simulink model "autosar_swc_monitor"  (R2021a)
settings: Solver=FixedStepDiscrete  StartTime=0.0  StopTime=10.0  FixedStep=0.02  RelTol=1e-3
PreLoadFcn:
  | Simulink.defineIntEnumType('SensorOption',...
  |     {'Primary', 'Secondary'},...
  |     [0;1],...
  |     'DefaultValue', 'Primary');
  | 
  | SensorSelection = Simulink.Parameter;
  | SensorSelection.Value = SensorOption.Primary;
  | SensorSelection.DataType = 'Enum: SensorOption';
libraries: simulink x1
settings Model: Creator=The MathWorks, Inc.  LastModifiedBy=ASUS
settings SolverCC: AlgebraicLoopSolver=TrustRegion
settings DataIOCC: SaveFormat=StructureWithTime  ReturnWorkspaceOutputs=off
settings OptimizationCC: DefaultParameterBehavior=Inlined  PassReuseOutputArgsAs=Individual arguments  ZeroExternalMemoryAtStartup=off  ZeroInternalMemoryAtStartup=off  EfficientTunableParamExpr=on
settings DebuggingCC: ParameterTunabilityLossMsg=error  SFMachineParentedDataDiag=warning  ArithmeticOperatorsInVariantConditions=warning
settings SFSimCC: SimUseLocalCustomCode=off  MATLABDynamicMemAlloc=off  CustomCodeUndefinedFunction=UseInterfaceOnly
settings RTWCC: Description=AUTOSAR  SystemTargetFile=autosar.tlc  GenCodeOnly=on  TemplateMakefile=ert_default_tmf  GenerateReport=on  RTWUseLocalCustomCode=off  IncludeHyperlinkInReport=on  LaunchReport=on  GenerateTraceInfo=on  GenerateTraceReport=on  GenerateTraceReportSl=on  GenerateTraceReportSf=on  GenerateTraceReportEml=on
settings CodeAppCC: ForceParamTrailComments=on  IgnoreCustomStorageClasses=off  OperatorAnnotations=on  SimulinkDataObjDesc=on  SFDataObjDesc=on  InsertBlockDesc=on
settings STFCustomTargetCC: TargetLangStandard=C99 (ISO)  MultiwordLength=256  ParMdlRefBuildCompliant=on  CompOptLevelCompliant=on  IncludeMdlTerminateFcn=off  CombineOutputUpdateFcns=on  SuppressErrorStatus=on  ERTCustomFileBanners=on  SupportNonFinite=off  SupportComplex=off  SupportContinuousTime=off  SupportNonInlinedSFcns=off  RemoveResetFunc=on  MATLABClassNameForMDSCustomization=Simulink.SoftwareTarget.ERTCustomization  AutosarCompliant=on  GRTInterface=off  LookupTableObjectStructAxisOrder=2,1,3,4,...  LUTObjectStructOrderEvenSpacing=Size,Table,Breakpoints  SystemTargetFile=autosar.tlc
settings ERTTargetCC: TargetLangStandard=C99 (ISO)  ConcurrentExecutionCompliant=off  IncludeMdlTerminateFcn=off  SuppressErrorStatus=on  SupportNonFinite=off  SupportComplex=off  ModelStepFunctionPrototypeControlCompliant=off  CPPClassGenCompliant=off  AutosarCompliant=on  LookupTableObjectStructAxisOrder=2,1,3,4,...  LUTObjectStructOrderEvenSpacing=Size,Table,Breakpoints  InlinedParameterPlacement=NonHierarchical  ERTCustomFileTemplate=example_file_process.tlc

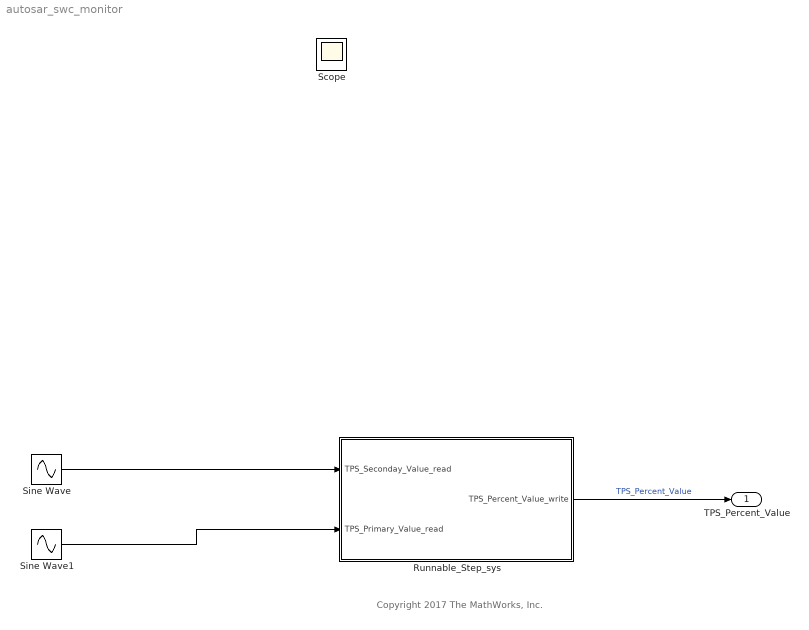
== system autosar_swc_monitor ==
  note: Copyright 2017 The MathWorks, Inc.
  Runnable_Step_sys : Subsystem  TreatAsAtomicUnit=on
  Sine Wave : Sin  SampleTime=0.02  VectorParams1D=off
  Sine Wave1 : Sin  SampleTime=0.02  VectorParams1D=off
  TPS_Percent_Value : Outport  PortDimensions=1  VectorParamsAs1DForOutWhenUnconnected=off
  Scope : Scope
  wires:
  Runnable_Step_sys/1(TPS_Percent_Value_write) -> TPS_Percent_Value/1  "TPS_Percent_Value"
  Sine Wave/1 -> Runnable_Step_sys/1(TPS_Seconday_Value_read)
  Sine Wave1/1 -> Runnable_Step_sys/2(TPS_Primary_Value_read)

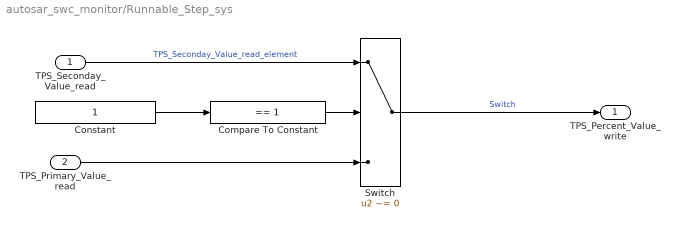
== system autosar_swc_monitor/Runnable_Step_sys ==
  TPS_Seconday_Value_read : Inport  SampleTime=0.02
  TPS_Primary_Value_read : Inport  Port=2  SampleTime=0.02
  Compare To Constant : simulink/Logic and Bit Operations/Compare To Constant  relop===  const=1  OutDataTypeStr=boolean
  Constant : Constant
  Switch : Switch  Criteria=u2 ~= 0
  TPS_Percent_Value_write : Outport  VectorParamsAs1DForOutWhenUnconnected=off
  wires:
  TPS_Seconday_Value_read/1 -> Switch/1  "TPS_Seconday_Value_read_element"
  TPS_Primary_Value_read/1 -> Switch/3
  Switch/1 -> TPS_Percent_Value_write/1  "Switch"
  Constant/1 -> Compare To Constant/1
  Compare To Constant/1 -> Switch/2
